simulink model "decision_frequency_error"  (R2014b)
settings: Solver=ode45  StartTime=0.0  StopTime=12000/fs  RelTol=1e-3
PreLoadFcn:
  | %%%%%%%%%%%%%%%%%%%%%%%%%%%%%%%%%%%%%%%%%%%%%%%%%%%%%%%%%%%%%%%%%%%%%%%%%%%
  | % check to see if Simulink library folder is missing from the MATLAB path %
  | %%%%%%%%%%%%%%%%%%%%%%%%%%%%%%%%%%%%%%%%%%%%%%%%%%%%%%%%%%%%%%%%%%%%%%%%%%%
  | if isempty(strfind(path, 'rtlsdr_book_library'))
  | 
  |     % create error window
  |     fig_error = figure(...
  |         'Name', 'Error: RTL-SDR Book Library',...
  |         'Toolbar','none',...
  |         'MenuBar','none',...
  |         'NumberTitle','off',...
  |         'Resize','off',...
  |         'WindowStyle','modal');
  |     fig_error.Position(3) = 600;
  |     fig_error.Position(4) = 150;
  |     fig_axes = axes(...
  |         'Parent',fig_error,...
  |         'Position',[0,0,1,1],...
  |         'visible','off');
  |     % error message
  |     t_title = text(.05,.8,...
  |         'MISSING DIRECTORIES',...
  |         'FontSize',11.5);
  |     t_body = text(.075,.6,...
  |         [{'Simulink cannot find the  \it{<root>}\rm / \it{rtlsdr\_book\_library}\rm  folder in the \it{MATLAB Path}\rm.'},...
  |         {'Please set the MATLAB path following the instructions given in Exercise 2.4.'}],...
  |         'FontSize',10.5);
  |     % buttons
  |     btn_path = uicontrol(...
  |         'Parent',fig_error,...
  |         'String','Set Path Now',...
  |         'FontSize',10,...
  |         'Callback', 'pathtool; close(fig_error);',...
  |         'Position', [fig_error.Position(3)/2-210, 30, 200, 30]);
  |     btn_abort = uicontrol(...
  |         'Parent',fig_error,...
  |         'String','No thanks',...
  |         'FontSize',10,...
  |         'Callback', 'close(fig_error); abort=1;',...
  |         'Position', [fig_error.Position(3)/2+10, 30, 200, 30]);
  | 
  |     % pause to allow user to interact with error box
  |     uiwait(fig_error);
  | 
  |     % abort simulation
  |     try
  |         if abort==1
  |             set_param(gcs, 'SimulationCommand', 'stop');
  |         end
  |     end
  | 
  |     % if user has set path, allow diagram to be updated
  |     if ~exist('abort','var')
  |         % create error window
  |         fig_update = figure(...
  |             'Name', 'Update Diagram',...
  |             'Toolbar','none',...
  |             'MenuBar','none',...
  |             'NumberTitle','off',...
  |             'Resize','off');
  |         fig_update.Position(3) = 400;
  |         fig_update.Position(4) = 120;
  |         fig_axes = axes(...
  |             'Parent',fig_update,...
  |             'Position',[0,0,1,1],...
  |             'visible','off');
  |         % instruction message
  |         t_body = text(.075,.7,...
  |             'Once you have set the path, update the block diagram',...
  |             'FontSize',10.5);
  |         % button
  |         btn_update = uicontrol(...
  |             'Parent',fig_update,...
  |             'String','Update Block Diagram',...
  |             'FontSize',10,...
  |             'Callback', 'set_param(gcs,''SimulationCommand'',''update''); close(gcf)',...
  |             'Position', [fig_update.Position(3)/2-100, 30, 200, 30]);
  |     end
  | 
  |     % clear error components
  |     clear('fig_error','fig_update','fig_axes','t_title','t_body','btn_path','btn_abort','btn_update','abort');
  | 
  | end
  | %%%%%%%%%%%%%%%%%%%%%%%%%%%%%%%%%%%%%%%%%%%%%%%%%%%%%%%%%%%%%%%%%%%%%%%%%%%
  | 
  | 
  | fs = 2.4e6;
  | MHz = fs/1e6;
  | 
  | 
  | Rdata = 100e3;
  | Rsymbol = Rdata/2;
  | interp = fs/Rsymbol;
  | 
  | 
  | % ---------------- synch loop design ------------------
  | 
  | d = 0.707;                 % damping ratio
  | 
  | Ts = 1/Rsymbol;         % symbol period
  | Ks = 0.5;                    % phase detector coefficientc
  | BnS = 0.02*Rsymbol;  % noise bandwidth in Hz
  | Kn   = 1;                     % gain of numerically controlled clock
  | 
  | % ------------ calculate loop filter coefficients -----------
  | 
  | Ka = (4*d*BnS*Ts)/(Kn*Ks*(d+1/(4*d)));
  | Kb = (4*(BnS*Ts)^2)/(Kn*Ks*(d+1/4*d)^2);
StopFcn:
  | % draw comparison of transmitted and received bits
  | 
  | tx_bits1 = squeeze(tx_bits);
  | rx_bits1 = squeeze(rx_bits);
  | 
  | len_tx = length(tx_bits1);
  | len_rx = length(rx_bits1);
  | max_len = max(len_tx, len_rx);
  | 
  | figure(3)
  | hold off
  | plot(tx_bits1,'r-x');
  | hold on
  | plot(rx_bits1,'b-o');
  | xlabel('Bit Index');
  | ylabel('Value');
  | axis([0 max_len -0.2 1.2]);
  | legend('Transmitted','Received','location','NorthEast');
  | grid on;
  | 
  | set(3,'Name','Comparison of Transmitted and Received Bits','NumberTitle','off');
  | setStandardFigSize(3);
undefined symbols (not defined in the file or in its folder): startfcn_constellation, startfcn_time_scope
libraries: commfilt2 x4, commdigbbndpm3 x2, dsparch4 x2, simulink x2, rtlsdr_book_library x1, commrandsrc2 x1
CloseFcn:
  | closefcn_model;
Description:
  | Software, Simulation Examples and Design Exercises Licence Agreement
  | 
  | This license agreement refers to the simulation examples, design exercises and files,
  | and associated software MATLAB and Simulink resources that accompany the book:
  | 
  |      Title: Software Defined Radio using MATLAB & Simulink and the RTL-SDR
  |      Published by Strathclyde Academic Media, 2015
  |      Authored by Robert W. Stewart, Kenneth W. Barlee, Dale S.W. Atkinson,
  |      and Louise H. Crockett
  | 
  | and made available as a download from, www.desktopSDR.com or variously acquired
  | by other means such as via USB storage, cloud storage, disk or any other electronic
  | or optical or magnetic storage mechanism. These files and associated software may
  | be used subject to the terms of agreement of the conditions below:
  | 
  |     Copyright © 2015 Robert W. Stewart, Kenneth W. Barlee, Dale S.W. Atkinson,
  |     and Louise H. Crockett
  |     All rights reserved.
  | 
  | Redistribution and use in source and binary forms, with or without modification, are
  | permitted provided that the following conditions are met:
  | 
  |    1.  Redistributions of source code must retain the above copyright notice, this list of
  |         conditions and the following disclaimer.
  | 
  |    2.  Redistributions in binary form must reproduce the above copyright notice, this
  |         list of conditions and the following disclaimer in the documentation and/or other
  |         materials provided with the distribution.
  | 
  |    3.  Neither the name of the copyright holder nor the names of its contributors may
  |         be used to endorse or promote products derived from this software without
  |         specific prior written permission.
  | 
  |    4.  In all cases, the software is, and all modifications and derivatives of the
  |         software shall be, licensed to you solely for use in conjunction with The
  |         MathWorks, Inc. products and service offerings.
  | 
  | THIS SOFTWARE IS PROVIDED BY THE COPYRIGHT HOLDERS AND CONTRIBUTORS
  | "AS IS" AND ANY EXPRESS OR IMPLIED WARRANTIES, INCLUDING, BUT NOT LIMITED
  | TO, THE IMPLIED WARRANTIES OF MERCHANTABILITY AND FITNESS FOR A
  | PARTICULAR PURPOSE ARE DISCLAIMED. IN NO EVENT SHALL THE COPYRIGHT
  | HOLDER OR CONTRIBUTORS BE LIABLE FOR ANY DIRECT, INDIRECT, INCIDENTAL,
  | SPECIAL, EXEMPLARY, OR CONSEQUENTIAL DAMAGES (INCLUDING, BUT NOT
  | LIMITED TO, PROCUREMENT OF SUBSTITUTE GOODS OR SERVICES; LOSS OF USE,
  | DATA, OR PROFITS; OR BUSINESS INTERRUPTION) HOWEVER CAUSED AND ON ANY
  | THEORY OF LIABILITY, WHETHER IN CONTRACT, STRICT LIABILITY, OR TORT
  | (INCLUDING NEGLIGENCE OR OTHERWISE) ARISING IN ANY WAY OUT OF THE USE
  | OF THIS SOFTWARE, EVEN IF ADVISED OF THE POSSIBILITY OF SUCH DAMAGE.
  | 
  | 
  | Audio Tracks used in Simulations Examples and Design Exercises
  | 
  | The music and vocal files used within the Examples files and software within the book
  | were variously written, arranged, performed, recorded and produced by Garrey Rice,
  | Adam Struth, Jamie Struth, Iain Thistlethwaite and also Marshall Craigmyle who
  | collectively, and individually where appropriate, assert and retain all of their copyright,
  | performance and artistic rights. Permission to use and reproduce this music is
  | granted for all purposes associated with MATLAB and Simulink software and the
  | simulation examples and design exercises files that accompany this book. Requests to
  | use the music for any other purpose should be directed to: info@desktopSDR.com.
  | For information on music track names, full credits, and links to the musicians please
  | refer to www.desktopSDR.com/more/audio.
settings Model: Creator=desktopSDR Team  LastModifiedBy=desktopSDR Team
settings OptimizationCC: UseDivisionForNetSlopeComputation=off  SimCompilerOptimization=off
settings DebuggingCC: FrameProcessingCompatibilityMsg=error
settings RTWCC: RTWCompilerOptimization=off

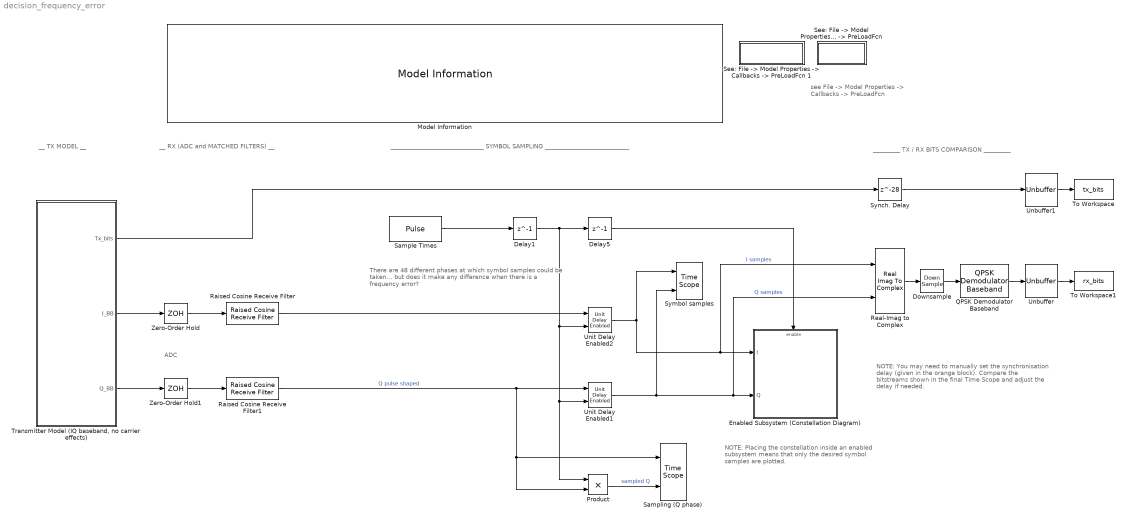
== system decision_frequency_error ==
  note: There are 48 different phases at which symbol
      | samples could be taken... but does it make any
      | difference when there is a frequency error?
  note: ADC
  note: NOTE:
      |
      | Placing the constellation inside an enabled
      | subsystem means that only the desired symbol
      | samples are plotted.
  note: _______________________________ SYMBOL SAMPLING ____________________________
  note: __ TX MODEL __
  note: __ RX (ADC and MATCHED FILTERS) __
  note: see File -> Model Properties
      | -> Callbacks -> PreLoadFcn
  note: _________ TX / RX BITS COMPARISON _________
  note: NOTE:
      |
      | You may need to manually set the synchronisation
      | delay (given in the orange block). Compare the
      | bitstreams shown in the final Time Scope and
      | adjust the delay if needed.
  Delay1 : Delay  DelayLength=1  SampleTime=1/fs
  Delay5 : Delay  DelayLength=1  SampleTime=1/fs
  Downsample : DownSample  N=48
  Enabled Subsystem (Constellation Diagram) : Subsystem  TreatAsAtomicUnit=on
  Model Information : rtlsdr_book_library/Additional Tools/Model Information/Model Information
  Product : Product
  QPSK Demodulator Baseband : commdigbbndpm3/QPSK Demodulator Baseband  Ph=pi/4  Dec=Gray  OutType=Bit  DecType=Hard decision  VarSource=Dialog  Variance=1  outDtype1=Inherit via internal rule  outDtype2=Inherit via internal rule  derotateFactorWordLen=16
  Raised Cosine Receive Filter : commfilt2/Raised Cosine Receive Filter  filtType=Square root  N=interp  filtSpan=12  currentFiltSpan=12  D=(12)/2  R=0.5  sampMode=Mute  saveAsFlag=0  rateMode=Downsampling  downFactor=1  downOffset=0  framing=Allow multirate processing  checkGain=Normalized  filterGain=1  checkCoeff=off  variableName=rcRxFilt1  launchFVT=on  roundingMode=Floor  overflowMode=off
  Raised Cosine Receive Filter1 : commfilt2/Raised Cosine Receive Filter  filtType=Square root  N=interp  filtSpan=12  currentFiltSpan=12  D=(12)/2  R=0.5  sampMode=Mute  saveAsFlag=0  rateMode=Downsampling  downFactor=1  downOffset=0  framing=Allow multirate processing  checkGain=Normalized  filterGain=1  checkCoeff=off  variableName=rcRxFilt  launchFVT=on  roundingMode=Floor  overflowMode=off
  Real-Imag to Complex : RealImagToComplex
  Sample Times : DiscretePulseGenerator  Period=interp  SampleTime=1/fs
  Sampling (Q phase) : TimeScope  StartFcn=startfcn_time_scope;  DefaultConfigurationName=spbscopes.TimeScopeBlockCfg  NumInputPorts=2
  "See: File -> Model Properties -> Callbacks -> PreLoadFcn " : Subsystem
      mask Display:
      | MHz = evalin('base', 'MHz');
      | fprintf(['fs = ',num2str(MHz),' MHz']);
  "See: File -> Model Properties -> Callbacks -> PreLoadFcn 1" : Subsystem
      mask Display:
      | Rdata = evalin('base', 'Rdata');
      | fprintf(['Rdata = ',num2str(Rdata/1e3),' ksps']);
  Symbol samples : TimeScope  StartFcn=startfcn_time_scope;  DefaultConfigurationName=spbscopes.TimeScopeBlockCfg  NumInputPorts=2
  Synch. Delay : Delay  DelayLength=28  InputProcessing=Columns as channels (frame based)
  To Workspace : ToWorkspace  VariableName=tx_bits  SampleTime=-1
  To Workspace1 : ToWorkspace  VariableName=rx_bits  SampleTime=-1
  "Transmitter Model (IQ baseband, no carrier effects)" : Subsystem  mask(Transmitter Model (Baseband Data)){Error=0.2}
      mask prompts: Error "% Timing Frequency Error"
      mask help: This transmitter block creates random QPSK data and applies RRC pulse shaping. The sample rate is adjusted based on the % timing frequency error specified in the mask. The outputs from the block are analogue I and Q channels.
      mask init:
      | Offset = 1+(Error/100);
  Unbuffer : Unbuffer  SampleBasedProcessing=Same as frame based
  Unbuffer1 : Unbuffer  SampleBasedProcessing=Same as frame based
  Unit Delay Enabled1 : simulink/Additional Math & Discrete/Additional Discrete/Unit Delay Enabled  vinit=0.0  tsamp=-1
  Unit Delay Enabled2 : simulink/Additional Math & Discrete/Additional Discrete/Unit Delay Enabled  vinit=0.0  tsamp=-1
  Zero-Order Hold : ZeroOrderHold  SampleTime=1/(Rsymbol*interp)
  Zero-Order Hold1 : ZeroOrderHold  SampleTime=1/(Rsymbol*interp)
  wires:
  "Transmitter Model (IQ baseband, no carrier effects)"/3(Q_BB) -> Zero-Order Hold1/1
  "Transmitter Model (IQ baseband, no carrier effects)"/2(I_BB) -> Zero-Order Hold/1
  Zero-Order Hold/1 -> Raised Cosine Receive Filter/1
  Zero-Order Hold1/1 -> Raised Cosine Receive Filter1/1
  Raised Cosine Receive Filter1/1 -> Unit Delay Enabled1/1, Sampling (Q phase)/1, Product/2  "Q pulse shaped"
  Raised Cosine Receive Filter/1 -> Unit Delay Enabled2/1
  Unit Delay Enabled2/1 -> Symbol samples/1, Real-Imag to Complex/1, Enabled Subsystem (Constellation Diagram)/1(I)  "I samples"
  Unit Delay Enabled1/1 -> Symbol samples/2, Real-Imag to Complex/2, Enabled Subsystem (Constellation Diagram)/2(Q)  "Q samples"
  Delay5/1 -> Enabled Subsystem (Constellation Diagram)/Enable
  Sample Times/1 -> Delay1/1
  Product/1 -> Sampling (Q phase)/2  "sampled Q"
  Delay1/1 -> Product/1, Unit Delay Enabled1/2, Unit Delay Enabled2/2, Delay5/1
  Downsample/1 -> QPSK Demodulator Baseband/1
  "Transmitter Model (IQ baseband, no carrier effects)"/1(Tx_bits) -> Synch. Delay/1
  QPSK Demodulator Baseband/1 -> Unbuffer/1
  Real-Imag to Complex/1 -> Downsample/1
  Unbuffer/1 -> To Workspace1/1
  Synch. Delay/1 -> Unbuffer1/1
  Unbuffer1/1 -> To Workspace/1

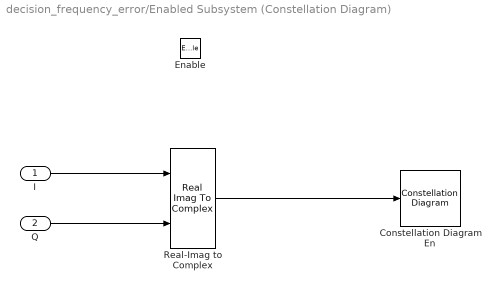
== system decision_frequency_error/Enabled Subsystem (Constellation Diagram) ==
  I : Inport
  Q : Inport  Port=2
  Enable : EnablePort
  Constellation Diagram En : ConstellationDiagram  StartFcn=startfcn_constellation;
  Real-Imag to Complex : RealImagToComplex
  wires:
  I/1 -> Real-Imag to Complex/1
  Q/1 -> Real-Imag to Complex/2
  Real-Imag to Complex/1 -> Constellation Diagram En/1

== system decision_frequency_error/See: File -> Model Properties -> Callbacks -> PreLoadFcn  ==

== system decision_frequency_error/See: File -> Model Properties -> Callbacks -> PreLoadFcn 1 ==

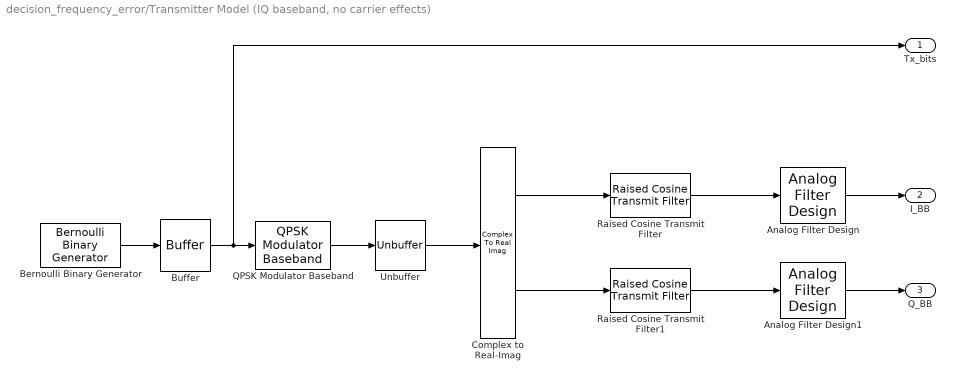
== system decision_frequency_error/Transmitter Model (IQ baseband, no carrier effects) ==
  Analog Filter Design : dsparch4/Analog Filter Design  method=Butterworth  filttype=Lowpass  N=8  Wlo=2*pi*Rsymbol*Offset  Whi=80  Rp=2  Rs=40
  Analog Filter Design1 : dsparch4/Analog Filter Design  method=Butterworth  filttype=Lowpass  N=8  Wlo=2*pi*Rsymbol*Offset  Whi=80  Rp=2  Rs=40
  Bernoulli Binary Generator : commrandsrc2/Bernoulli Binary Generator  P=0.5  seed=610  Ts=1/(Offset*Rdata)  frameBased=off  sampPerFrame=2  orient=on  outDataType=double
  Buffer : Buffer  N=2  TreatMby1Signals=One channel
  Complex to Real-Imag : ComplexToRealImag
  QPSK Modulator Baseband : commdigbbndpm3/QPSK Modulator Baseband  InType=Bit  Enc=Gray  Ph=pi/4  outDtype=double  outWordLen=16  outUDDataType=sfix(16)  outFracLenMode=Best precision  outFracLen=15
  Raised Cosine Transmit Filter : commfilt2/Raised Cosine Transmit Filter  filtType=Square root  filtSpan=12  currentFiltSpan=12  D=(12)/2  R=0.5  sampMode=Mute  saveAsFlag=0  N=interp  framing=Allow multirate processing  checkGain=Normalized  filterGain=1  checkCoeff=off  variableName=rcTxFilt  launchFVT=on  roundingMode=Floor  overflowMode=off
  Raised Cosine Transmit Filter1 : commfilt2/Raised Cosine Transmit Filter  filtType=Square root  filtSpan=12  currentFiltSpan=12  D=(12)/2  R=0.5  sampMode=Mute  saveAsFlag=0  N=interp  framing=Allow multirate processing  checkGain=Normalized  filterGain=1  checkCoeff=off  variableName=rcTxFilt1  launchFVT=on  roundingMode=Floor  overflowMode=off
  Unbuffer : Unbuffer  SampleBasedProcessing=Same as frame based
  Tx_bits : Outport
  I_BB : Outport  Port=2
  Q_BB : Outport  Port=3
  wires:
  Raised Cosine Transmit Filter1/1 -> Analog Filter Design1/1
  Unbuffer/1 -> Complex to Real-Imag/1
  Complex to Real-Imag/2 -> Raised Cosine Transmit Filter1/1
  Complex to Real-Imag/1 -> Raised Cosine Transmit Filter/1
  QPSK Modulator Baseband/1 -> Unbuffer/1
  Analog Filter Design1/1 -> Q_BB/1
  Analog Filter Design/1 -> I_BB/1
  Raised Cosine Transmit Filter/1 -> Analog Filter Design/1
  Bernoulli Binary Generator/1 -> Buffer/1
  Buffer/1 -> Tx_bits/1, QPSK Modulator Baseband/1
